simulink model "Epidemic Spread Analysis SIMULINK"  (R2022a)
settings: Solver=VariableStepAuto  StartTime=0.0  StopTime=50  RelTol=1e-3
settings Model: Creator=nathan  LastModifiedBy=nathan

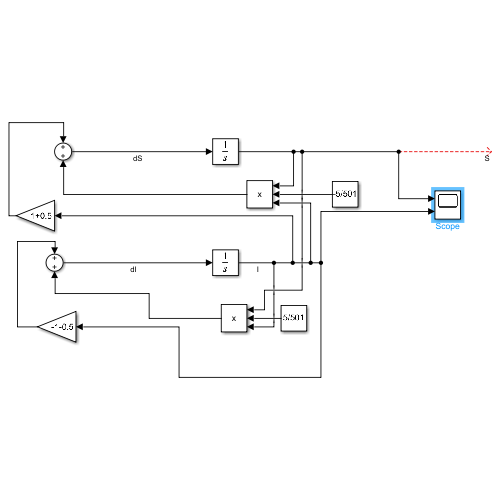
[thumbnail: Simulink's stored preview of the top-level diagram]
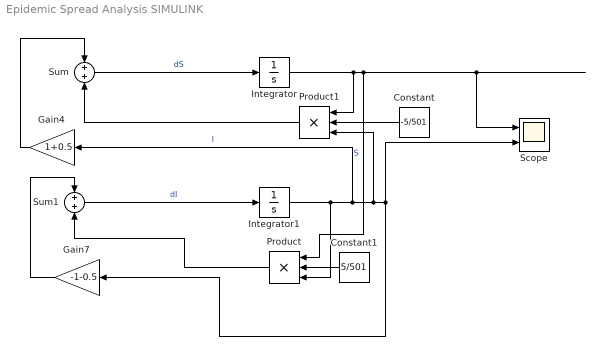
== system Epidemic Spread Analysis SIMULINK ==
  Constant : Constant  Value=-5/501
  Constant1 : Constant  Value=5/501
  Gain4 : Gain  Gain=1+0.5
  Gain7 : Gain  Gain=-1-0.5
  Integrator : Integrator  InitialCondition=500
  Integrator1 : Integrator  InitialCondition=1
  Product : Product  Inputs=3
  Product1 : Product  Inputs=3
  Scope : Scope  NumInputPorts=2
  Sum : Sum
  Sum1 : Sum
  wires:
  Sum/1 -> Integrator/1  "dS"
  Integrator/1 -> Product1/1, Scope/1, Product/1  "S"
  Integrator1/1 -> Product/3, Product1/3, Scope/2, Gain7/1, Gain4/1  "I"
  Sum1/1 -> Integrator1/1  "dI"
  Gain4/1 -> Sum/1
  Gain7/1 -> Sum1/1
  Constant/1 -> Product1/2
  Product1/1 -> Sum/2
  Constant1/1 -> Product/2
  Product/1 -> Sum1/2
